simulink library "RIFFTLib"  (R2022b)
settings: Solver=VariableStepAuto  StartTime=0.0  StopTime=10.0  RelTol=1e-3
settings Model: Creator=ud1041536  LastModifiedBy=kl13806
settings SolverCC: AlgebraicLoopSolver=TrustRegion
settings DebuggingCC: UnconnectedInputMsg=warning  UnconnectedOutputMsg=warning  UnconnectedLineMsg=warning  SFMachineParentedDataDiag=warning  ArithmeticOperatorsInVariantConditions=warning
settings ModelReferenceCC: EnableRefExpFcnMdlSchedulingChecks=on
settings SFSimCC: CustomCodeUndefinedFunction=UseInterfaceOnly
settings RTWCC: DLArmComputeVersion=19.05

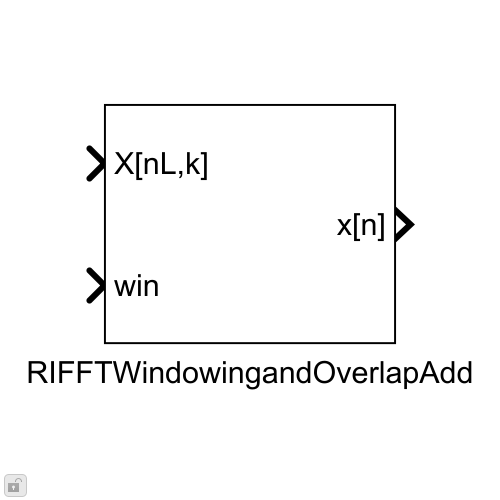
[thumbnail: Simulink's stored preview of the top-level diagram]
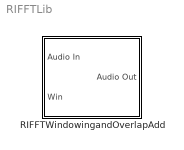
== system RIFFTLib ==
  RIFFTWindowingandOverlapAdd : Subsystem  mask(Real IFFT with Windowing and Overlap-Add){variantSelect=Core, fftSize=256, numOverlap=128, bufferAlias=default}
      mask prompts: variantSelect "Implementation:"; fftSize "FFT size"; numOverlap "Number of overlapping samples:"; bufferAlias "Alias (must be unique across all instances in model)"
      mask help:
      | This block computes the Inverse Fourier Transform using an optimized IFFT for complex half-spectra, followed by in-place windowing and overlap-add. It only supports even number of channels, and 128-point or 256-point FFT.
      |
      | 2 current implementation types are:
      | (i) Core
      | (ii) Generic
      mask init:
      | RifftMaskInit(gcbh, fftSize, bufferAlias, variantSelect)
      mask TypeOptions variantSelect: Core | Generic
      mask Display:
      | port_label('output',1,'x[n]')
      | port_label('input',1,'X[nL,k]')
      | port_label('input',2,'win')

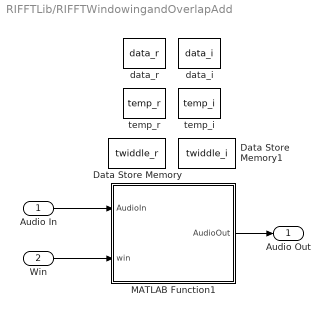
== system RIFFTLib/RIFFTWindowingandOverlapAdd ==
  Audio In : Inport
  Win : Inport  Port=2
  Data Store Memory : DataStoreMemory  DataStoreName=twiddle_r  ReadBeforeWriteMsg=warning  WriteAfterWriteMsg=warning  WriteAfterReadMsg=warning  ShowAdditionalParam=off  OutDataTypeStr=uint32
  Data Store Memory1 : DataStoreMemory  DataStoreName=twiddle_i  ReadBeforeWriteMsg=warning  WriteAfterWriteMsg=warning  WriteAfterReadMsg=warning  ShowAdditionalParam=off  OutDataTypeStr=uint32
  MATLAB Function1 : MATLAB Function  TreatAsAtomicUnit=on
  data_i : DataStoreMemory  DataStoreName=data_i  ReadBeforeWriteMsg=warning  WriteAfterWriteMsg=warning  WriteAfterReadMsg=warning  InitialValue=zeros(fftSize,1)  EmbeddedSignalClassName=Blocklib.Signal  ShowAdditionalParam=off  OutDataTypeStr=single
  data_r : DataStoreMemory  DataStoreName=data_r  ReadBeforeWriteMsg=warning  WriteAfterWriteMsg=warning  WriteAfterReadMsg=warning  InitialValue=zeros(fftSize,1)  EmbeddedSignalClassName=Blocklib.Signal  ShowAdditionalParam=off  OutDataTypeStr=single
  temp_i : DataStoreMemory  DataStoreName=temp_i  ReadBeforeWriteMsg=warning  WriteAfterWriteMsg=warning  WriteAfterReadMsg=warning  InitialValue=zeros(fftSize,1)  EmbeddedSignalClassName=Blocklib.Signal  ShowAdditionalParam=off  OutDataTypeStr=single
  temp_r : DataStoreMemory  DataStoreName=temp_r  ReadBeforeWriteMsg=warning  WriteAfterWriteMsg=warning  WriteAfterReadMsg=warning  InitialValue=zeros(fftSize,1)  EmbeddedSignalClassName=Blocklib.Signal  ShowAdditionalParam=off  OutDataTypeStr=single
  Audio Out : Outport  VectorParamsAs1DForOutWhenUnconnected=off
  wires:
  Audio In/1 -> MATLAB Function1/1(AudioIn)
  MATLAB Function1/1(AudioOut) -> Audio Out/1
  Win/1 -> MATLAB Function1/2(win)

== matlab function RIFFTLib/RIFFTWindowingandOverlapAdd/MATLAB Function1 ==
  data: AudioIn input; AudioOut output; fftSize parameter; numOverlap parameter; win input; data_r data_store_memory; data_i data_store_memory; temp_r data_store_memory; temp_i data_store_memory; twiddle_r data_store_memory; twiddle_i data_store_memory; variantSelect parameter
function AudioOut = ifftReal(AudioIn, fftSize, numOverlap, win, variantSelect)   

global data_r
global data_i
global temp_r
global temp_i
global twiddle_r
global twiddle_i

[~, numChannels] = size(AudioIn);
outputSize = fftSize - numOverlap;

% Buffer to hold overlapped samples
persistent outputOverlap;
if isempty(outputOverlap)
    outputOverlap = single(zeros(numOverlap, numChannels));
end

% Nullcopy copies type, size, and complexity of input to output
AudioOut = coder.nullcopy(single(zeros(outputSize, numChannels)));

% Set correct data types
fftSize = uint32(fftSize);
numChannels = uint32(numChannels);
numOverlap = uint32(numOverlap);

% There are two implementation types:
% Type    Value   Description
% CORE    1       Optimized assembly running on SHARC+ core
% GENERIC 2       Generic implementation for other targets without CRL

% Simulation
if(coder.target('MATLAB') || coder.target('Sfun')) 
   AudioOut = rifft_simulation(AudioIn, win, numOverlap);       
    
% Code generation
else
    % Core
    if (variantSelect == 1) 
        % Set the twiddle pointers to correct twiddle table
        % The pointers are of type uint32 here and will be casted to float* 
        % in the code-replaced function. The twiddle tables are declared in 
        % a separate file and will be pulled in through CRL.
        if fftSize == 256
            coder.ceval('set_twiddle_256', coder.wref(twiddle_r), coder.wref(twiddle_i));
        else
            coder.ceval('set_twiddle_128', coder.wref(twiddle_r), coder.wref(twiddle_i));
        end
        AudioOut = rifft_process(AudioIn, data_r, data_i, temp_r, temp_i, win, ...
            outputOverlap, twiddle_r, twiddle_i, fftSize, numChannels, numOverlap);
        
    % Generic
    else
        AudioOut = rifft_simulation(AudioIn, win, numOverlap);       
    end
end

end    

%% CRL function for code generation
function y = rifft_process(u, data_r, data_i, temp_r, temp_i, win, ...
    output_overlap, twiddle_r, twiddle_i, fft_size, num_channel, num_overlap)
% If target == codegen, error out if no CRL found
coder.replace('-errorifnoreplacement'); 
y = (single(zeros(fft_size - num_overlap, num_channel)));

end

%% Function for simulation
function y = rifft_simulation(u, win, num_overlap)

% Restore conjugate symmetry
newPart = u(2:end-1, :);         % Get N-2 middle points 
newPart = flipud(conj(newPart)); % Conjugate and flip
y = [u; newPart];                % Concat to get full spectrum

% Perform ifft
y = ifft(y); 

% Window and overlap-add
% Note: This function creates another outputOverlap buffer since Matlab
% variables can only be passed by value
y = winOverlapAdd(y, win, num_overlap);

end

function y = winOverlapAdd(u, win, numOverlap)

% Get sizes
[N, numChannels] = size(u);
L = N - numOverlap;

% Buffer to hold overlapped samples
persistent lastFrame;
if isempty(lastFrame)
    lastFrame = single(zeros(numOverlap, numChannels));
end

% Cast to real and apply window
% Loop since array-vector multiply operation doesn't work here
u = real(u);
for i = 1:numChannels
    u(:, i) = u(:,i) .* win;
end

% Overlap and add
u(1:numOverlap,:) = u(1:numOverlap,:) + lastFrame;

% Output first L samples
y = u(1:L, :); 

% Update buffer with the other N-L samples
lastFrame = u(L+1: end, :);

end
